simulink model "Lab4"  (R2022a)
settings: Solver=ode23t  StartTime=0.0  StopTime=3  MaxStep=1e-4  RelTol=1e-3
values from neighbouring files (symbols this model uses):
  f_1 = 50    [Lab4.m]
  J = 0.2    [Lab4.m]
  K2 = Lm/L2    (= 0.953488372093)    [Lab4.m]
  L_1 = L1*(1-K1*K2)    (= 0.0126279069767)    [Lab4.m]
  Llr = L2-Lm    (= 0.008)    [Lab4.m]
  Lls = L1-Lm    (= 0.005)    [Lab4.m]
  Pn = 5500    [Lab4.m]
  R1 = 1.32    [Lab4.m]
  R2 = 0.92    [Lab4.m]
  R_1 = (K2^2)*R2+R1    (= 2.15640886966)    [Lab4.m]
  T2 = L2/R2    (= 0.186956521739)    [Lab4.m]
  T_1 = L_1/R_1    (= 0.00585598916533)    [Lab4.m]
  Tn = Pn*z/((1-s_n)*2*pi*f_1)    (= 36.2840284769)    [Lab4.m]
  U_l = sqrt(3)*U_m    [Lab4.m]
  U_m = 220    [Lab4.m]
  w0 = 2*pi*f_1/z    (= 157.079632679)    [Lab4.m]
  z = 2    [Lab4.m]
libraries: mcbcontrolslib x4, spsControlledVoltageSourceLib x3, autolibim x2, spsAsynchronousMachineSIUnitsLib x1, spsGroundLib x1, spsThreePhaseVIMeasurementLib x1, simulink x1, spspowerguiLib x1
settings Model: Creator=hdu  LastModifiedBy=81502

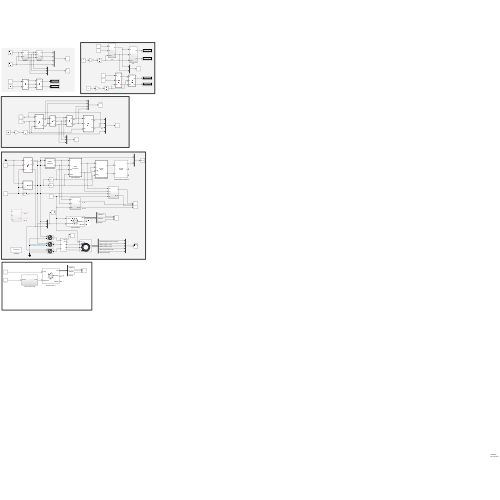
[thumbnail: Simulink's stored preview of the top-level diagram]
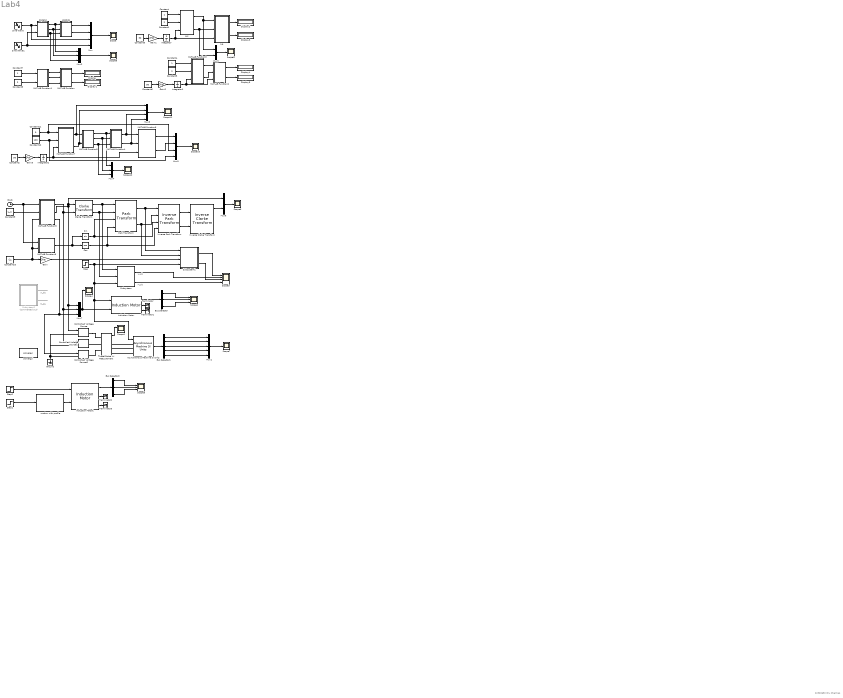
== system Lab4 ==
  note: 22320630
      | Zhu Chenhao
  note: w_ab
  note: M_ab
  note: w_dq
  note: M_dq
  Asynchronous Machine SI Units : spsAsynchronousMachineSIUnitsLib/Asynchronous Machine SI Units  RotorType=Squirrel-cage  PresetModel=No  MechanicalLoad=Torque Tm  ShowDetailedParameters=on  ReferenceFrame=Stationary  Units=SI  MeasurementBus=off  NominalParameters=[Pn U_l f_1]  VoltageRatio=1  Stator=[R1 Lls]  Rotor=[R2 Llr]  Cage1=[0.4155 0.002066]  Cage2=[0.4168 0.0003495]  Lm=Lm  Mechanical=[J 0.005752 z]  PolePairs=2  InitialConditions=[1 0 0 0 0 0 0 0]  SimulateSaturation=off  Saturation=[14.03593122, 27.81365428, 53.79336849, 72.68890987, 97.98006896, 148.6815601, 215.7428561, 302.9841135, 428.7778367 ; 230, 322, 414, 460, 506, 552, 598, 644, 690]  LoadFlowParameters=1492000  TsPowergui=0  TsBlock=-1  IterativeModel=Trapezoidal non iterative  IterativeDiscreteModel=Trapezoidal non iterative  Pmec=0
  Bus Selector : BusSelector  OutputSignals=IaStator,MtrSpd,MtrTrq
  Bus Selector1 : BusSelector  OutputSignals=Mechanical.Electromagnetic torque Te (N*m),Stator measurements.Stator current is_b (A),Stator measurements.Stator current is_a (A),Mechanical.Rotor angle thetam (rad),Mechanical.Rotor speed (wm)
  Bus Selector2 : BusSelector  OutputSignals=IaStator,MtrSpd,MtrTrq
  Clarke Transform : mcbcontrolslib/Clarke Transform  VariantControl=Variant2
  Clock : Clock
  Constant : Constant
  Constant1 : Constant  Value=2
  Constant10 : Constant  Value=f_1
  Constant11 : Constant  Value=0
  Constant12 : Constant  Value=100
  Constant2 : Constant  Value=50
  Constant3 : Constant  Value=50
  Constant4 : Constant
  Constant5 : Constant  Value=2
  Constant6 : Constant  Value=50
  Constant7 : Constant
  Constant8 : Constant  Value=2
  Constant9 : Constant  Value=U_m
  Controlled Voltage Source : spsControlledVoltageSourceLib/Controlled Voltage Source  Initialize=off  Source_Type=AC  Amplitude=0  Phase=0  Frequency=0  Measurements=None
  Controlled Voltage Source1 : spsControlledVoltageSourceLib/Controlled Voltage Source  Initialize=off  Source_Type=AC  Amplitude=0  Phase=0  Frequency=0  Measurements=None
  Controlled Voltage Source2 : spsControlledVoltageSourceLib/Controlled Voltage Source  Initialize=off  Source_Type=AC  Amplitude=0  Phase=0  Frequency=0  Measurements=None
  Cos : Trigonometry  Operator=cos
  Display{,1..5} (6 alike) : Display
  Gain{,1..3} (4 alike) : Gain  Gain=2*pi
  Ground : spsGroundLib/Ground  LConnTagsString=a
  Induction Motor : autolibim/Induction Motor  sim_type=Continuous  Ts=0.001  port_config=Torque  P=z  Zs=[R1 Lls]  Zr=[R2 Llr]  Lm=Lm  mechanical=[J 0 0]  theta_init=0  omega_init=0  RefBlkName='autolibim/Induction Motor'  aMode=1
      settings: SourceProductBaseCode=PW,DR,MT,VE
  Induction Motor1 : autolibim/Induction Motor  sim_type=Continuous  Ts=0.001  port_config=Torque  P=z  Zs=[R1 Lls]  Zr=[R2 Llr]  Lm=Lm  mechanical=[J 0 0]  theta_init=0  omega_init=0  RefBlkName='autolibim/Induction Motor'  aMode=1
      settings: SourceProductBaseCode=PW,DR,MT,VE
  Integrator : Integrator
  Integrator1 : Integrator
  Integrator2 : Integrator
  Inverse Clarke Transform : mcbcontrolslib/Inverse Clarke Transform
      settings: SourceProductBaseCode=MT
  Inverse Park Transform : mcbcontrolslib/Inverse Park Transform  AxisAlignment=D-axis
  MATLAB Function : MATLAB Function  TreatAsAtomicUnit=on
  MATLAB Function1 : MATLAB Function  TreatAsAtomicUnit=on
  MATLAB Function2 : MATLAB Function  TreatAsAtomicUnit=on
  MATLAB Function3 : MATLAB Function  TreatAsAtomicUnit=on
  MATLAB Function4 : MATLAB Function  TreatAsAtomicUnit=on
  MATLAB Function5 : MATLAB Function  TreatAsAtomicUnit=on
  MATLAB Function6 : MATLAB Function  TreatAsAtomicUnit=on
  MATLAB Function7 : MATLAB Function  TreatAsAtomicUnit=on
  MATLAB Function8 : MATLAB Function  TreatAsAtomicUnit=on
  MATLAB Function9 : MATLAB Function  TreatAsAtomicUnit=on
  Mux : Mux
  Mux1 : Mux  Inputs=5
  Mux2 : Mux  Inputs=3
  Mux3 : Mux  Inputs=2
  Mux4 : Mux  Inputs=3
  Mux5 : Mux
  Mux6 : Mux  Inputs=2
  Mux7 : Mux  Inputs=3
  Mux8 : Mux
  Park Transform : mcbcontrolslib/Park Transform  AxisAlignment=D-axis
      settings: SourceProductBaseCode=MT
  Scope{,4,6..12} (9 alike) : Scope
  Scope1 : Scope  NumInputPorts=2
  Scope2 : Scope  NumInputPorts=3
  Scope3 : Scope  NumInputPorts=4
  Scope5 : Scope  NumInputPorts=3
  Sin : Trigonometry
  Sine Wave : Sin  Amplitude=310  Frequency=2*pi*50  SampleTime=0
  Sine Wave1 : Sin  Amplitude=310  Frequency=2*pi*50  Phase=pi/2  SampleTime=0
  Step : Step  After=Tn  SampleTime=0
  Step1 : Step  Time=0.1  After=200  SampleTime=0
  Step2 : Step  Time=3  After=Tn  SampleTime=0
  Subsystem : Subsystem
  Subsystem1 : Subsystem
  Subsystem2 : Subsystem  Commented=on
  Terminator{,1..3} (4 alike) : Terminator
  Three-Phase V-I Measurement : spsThreePhaseVIMeasurementLib/Three-Phase V-I Measurement  VoltageMeasurement=phase-to-ground  SetLabelV=off  LabelV=Vabc  Vpu=off  VpuLL=off  CurrentMeasurement=yes  SetLabelI=off  LabelI=Iabc  Ipu=off  Pbase=100e6  Vbase=500e3  OutputType=Complex  PhasorSimulation=off  PSBequivalent=0
  abc2dp : Subsystem
  dq2abc : Subsystem
  e-s : Subsystem
  motion with profile : Subsystem
  powergui : spspowerguiLib/powergui  Priority=1  SimulationMode=Continuous  SampleTime=50e-6  frequency=60  Iterations=50  frequencyindice=50  Pbase=100e6  ErrMax=1e-4  UnitsV=kV  UnitsW=MW  buscounter=0  FunctionMessages=off  echomessages=off  EnableUseOfTLC=off  CurrentSourceSwitches=off  DisableSnubberDevices=off  DisableRonSwitches=off  DisableVfSwitches=off  DisplayEquations=off  AutomaticDiscreteSolvers=off  SolverType=Tustin/Backward Euler (TBE)  Interpol=off  ExternalGateDelay=off  methode=off  Ts=100  x0status=blocks  SPID=on  SwTol=0  HookPort=off  NonlinearTolerance=1e-4  nMaxIteration=100  ContinueOnMaxIteration=off  RestoreLinks=warning  ResistiveCurrentMeasurement=off  Frange=[0:2:500]  Ylog=off  Xlog=on  ShowGrid=off  save=off  variable=ZData  structure=0  ZoomFFT=off  StartTime=0.0  cycles=1  DisplayStyle=1  fundamental=60  FreqAxis=off  MaxFrequency=1000  frequencyindicesteady=1  RmsSteady=1  display=off
  s-e : Subsystem
  wires:
  Constant10/1 -> MATLAB Function9/3(f_1), MATLAB Function8/2(f_1), Gain/1
  Clock/1 -> MATLAB Function8/1(t), MATLAB Function9/1(t)
  MATLAB Function8/1(theta) -> Sin/1, Cos/1
  Constant9/1 -> MATLAB Function9/2(A)
  MATLAB Function9/2(ub) -> Mux6/1, Clarke Transform/1, Controlled Voltage Source/1, Mux7/1
  MATLAB Function9/1(ua) -> Clarke Transform/2, Mux7/2, Controlled Voltage Source1/1
  Clarke Transform/1 -> Park Transform/1, Subsystem/1(Ua)
  Clarke Transform/2 -> Subsystem/2(Ub), Park Transform/2
  Sin/1 -> Park Transform/3, Inverse Park Transform/3
  Cos/1 -> Park Transform/4, Inverse Park Transform/4
  Park Transform/2 -> Inverse Park Transform/2, Subsystem1/2(Uq)
  Park Transform/1 -> Inverse Park Transform/1, Subsystem1/1(Ud)
  Step/1 -> Asynchronous Machine SI Units/1, Induction Motor/1, Subsystem/3(Mc), Subsystem1/4(Mc)
  Inverse Park Transform/2 -> Inverse Clarke Transform/2
  Inverse Park Transform/1 -> Inverse Clarke Transform/1
  Inverse Clarke Transform/1 -> Mux6/2
  MATLAB Function9/3(uc) -> Controlled Voltage Source2/1, Mux7/3
  Mux7/1 -> Scope4/1, Induction Motor/2
  Mux6/1 -> Scope6/1
  Induction Motor/2 -> Terminator/1
  Induction Motor/1 -> Bus Selector/1
  Bus Selector/1 -> Scope2/1  "<IaStator>"
  Bus Selector/2 -> Scope2/2  "<MtrSpd>"
  Bus Selector/3 -> Scope2/3  "<MtrTrq>"
  Subsystem/1(w) -> Scope3/2
  Subsystem/2(M din) -> Scope3/4
  Asynchronous Machine SI Units/1 -> Bus Selector1/1
  Bus Selector1/1 -> Mux1/1  "<Electromagnetic torque Te (N*m)>"
  Bus Selector1/3 -> Mux1/3  "<Stator current is_a (A)>"
  Bus Selector1/4 -> Mux1/4  "<Rotor angle thetam (rad)>"
  Bus Selector1/5 -> Mux1/5  "<Rotor speed (wm)>"
  Bus Selector1/2 -> Mux1/2  "<Stator current is_b (A)>"
  Mux1/1 -> Scope7/1
  Gain/1 -> Subsystem1/3(w1)
  Subsystem1/1(w) -> Scope3/1
  Subsystem1/2(M din) -> Scope3/3
  Three-Phase V-I Measurement/1 -> Scope1/1
  Subsystem2/2(M din) -> ?
  Subsystem2/1(w) -> ?
  Induction Motor/3 -> Terminator1/1
  Induction Motor1/3 -> Terminator3/1
  Bus Selector2/3 -> Scope5/3  "<MtrTrq>"
  Induction Motor1/2 -> Terminator2/1
  Induction Motor1/1 -> Bus Selector2/1
  Bus Selector2/1 -> Scope5/1  "<IaStator>"
  Bus Selector2/2 -> Scope5/2  "<MtrSpd>"
  Step2/1 -> Induction Motor1/1
  Mux5/1 -> Scope10/1
  Constant6/1 -> Gain2/1
  Constant2/1 -> Gain3/1
  e-s/2(qs) -> Mux3/2, s-e/2(qs)
  Mux2/1 -> Scope8/1
  Mux8/1 -> Scope11/1
  Constant4/1 -> MATLAB Function3/1(de)
  Gain3/1 -> Integrator2/1
  MATLAB Function6/1(de) -> Mux5/1  "de"
  MATLAB Function7/2(qs) -> Mux8/2, MATLAB Function5/2(qs)  "qs"
  MATLAB Function1/1(a) -> MATLAB Function/1(a)
  e-s/1(ds) -> Mux3/1, s-e/1(ds)
  Constant3/1 -> Gain1/1
  MATLAB Function4/2(qs) -> Mux8/4, MATLAB Function6/2(qs)  "qs1"
  Mux3/1 -> Scope9/1
  MATLAB Function7/1(ds) -> Mux8/1, MATLAB Function5/1(ds)  "ds"
  MATLAB Function4/1(ds) -> Mux8/3, MATLAB Function6/1(ds)  "ds1"
  Integrator/1 -> s-e/3(theta), e-s/3(theta)
  Constant11/1 -> Mux5/3, MATLAB Function7/1(de)  "de"
  MATLAB Function3/1(ds) -> MATLAB Function2/1(ds)
  dq2abc/3(c) -> abc2dp/3(c), Mux2/3
  Mux4/1 -> Scope12/1
  abc2dp/2(qs) -> Mux/2
  MATLAB Function/2(qs) -> Display1/1
  Constant7/1 -> MATLAB Function1/1(ds)
  MATLAB Function1/3(c) -> MATLAB Function/3(c)
  Constant8/1 -> MATLAB Function1/2(qs)
  Sine Wave1/1 -> dq2abc/2(qs), Mux/4
  Integrator1/1 -> MATLAB Function2/3(teta), MATLAB Function3/3(teta)
  MATLAB Function2/2(qe) -> Display5/1
  MATLAB Function3/2(qs) -> MATLAB Function2/2(qs)
  Constant12/1 -> Mux5/4, MATLAB Function7/2(qe)  "qe"
  MATLAB Function1/2(b) -> MATLAB Function/2(b)
  Gain2/1 -> Integrator1/1
  MATLAB Function6/2(qe) -> Mux5/2  "dq"
  Gain1/1 -> Integrator/1
  MATLAB Function5/2(b) -> Mux4/2, MATLAB Function4/2(b)  "b"
  Mux/1 -> Scope/1
  s-e/2(qe) -> Display3/1
  MATLAB Function5/1(a) -> Mux4/1, MATLAB Function4/1(a)  "a"
  Integrator2/1 -> MATLAB Function6/3(teta), MATLAB Function7/3(teta)
  s-e/1(de) -> Display2/1
  Constant1/1 -> e-s/2(qe)
  Sine Wave/1 -> Mux/3, dq2abc/1(ds)
  MATLAB Function/1(ds) -> Display/1
  Constant/1 -> e-s/1(de)
  MATLAB Function2/1(de) -> Display4/1
  abc2dp/1(ds) -> Mux/1
  Constant5/1 -> MATLAB Function3/2(qe)
  dq2abc/1(a) -> Mux2/1, abc2dp/1(a)
  MATLAB Function5/3(c) -> Mux4/3, MATLAB Function4/3(c)  "c"
  dq2abc/2(b) -> Mux2/2, abc2dp/2(b)
  Step1/1 -> motion with profile/1(Speed)
  motion with profile/1(Vabc) -> Induction Motor1/2
  connections:
  Ground/LConn1 -- Controlled Voltage Source/LConn1 -- Controlled Voltage Source1/LConn1 -- Controlled Voltage Source2/LConn1
  Three-Phase V-I Measurement/LConn2 -- Controlled Voltage Source1/RConn1
  Controlled Voltage Source/RConn1 -- Three-Phase V-I Measurement/LConn1
  Three-Phase V-I Measurement/LConn3 -- Controlled Voltage Source2/RConn1
  Asynchronous Machine SI Units/LConn1 -- Three-Phase V-I Measurement/RConn1
  Asynchronous Machine SI Units/LConn2 -- Three-Phase V-I Measurement/RConn2
  Asynchronous Machine SI Units/LConn3 -- Three-Phase V-I Measurement/RConn3

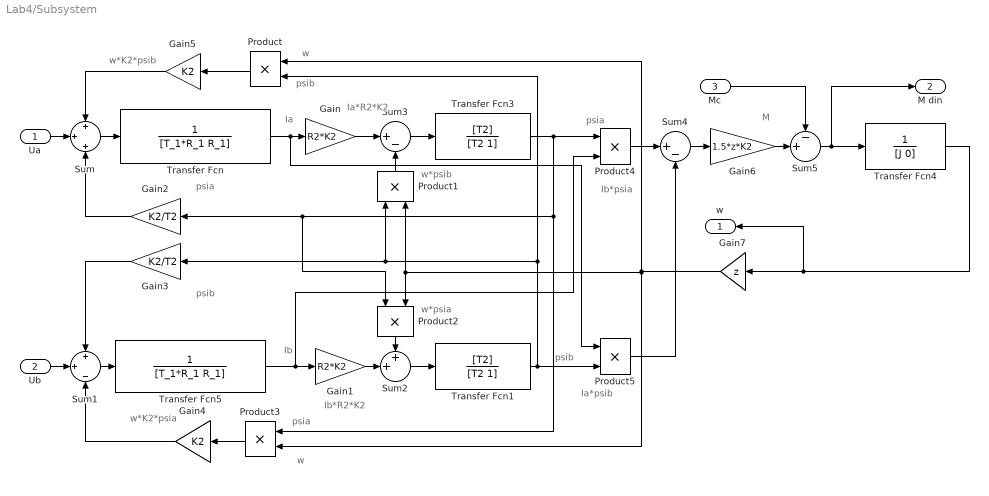
== system Lab4/Subsystem ==
  note: Ia*psib
  note: psib
  note: w
  note: psia
  note: w
  note: psib
  note: w*psia
  note: M
  note: Ib*psia
  note: psia
  note: w*psib
  note: Ib
  note: psib
  note: psia
  note: Ia
  note: w*K2*psib
  note: w*K2*psia
  note: Ia*R2*K2
  note: Ib*R2*K2
  Ua : Inport
  Ub : Inport  Port=2
  Mc : Inport  Port=3
  Gain : Gain  Gain=R2*K2
  Gain1 : Gain  Gain=R2*K2
  Gain2 : Gain  Gain=K2/T2
  Gain3 : Gain  Gain=K2/T2
  Gain4 : Gain  Gain=K2
  Gain5 : Gain  Gain=K2
  Gain6 : Gain  Gain=1.5*z*K2
  Gain7 : Gain  Gain=z
  Product{,1..5} (6 alike) : Product
  Sum : Sum  Inputs=+|+|+
  Sum1 : Sum  Inputs=+|+|-
  Sum2 : Sum  Inputs=++|
  Sum3 : Sum  Inputs=|+-
  Sum4 : Sum  Inputs=|+-
  Sum5 : Sum  Inputs=-+|
  Transfer Fcn : TransferFcn  Denominator=[T_1*R_1 R_1]
  Transfer Fcn1 : TransferFcn  Numerator=[T2]  Denominator=[T2 1]
  Transfer Fcn3 : TransferFcn  Numerator=[T2]  Denominator=[T2 1]
  Transfer Fcn4 : TransferFcn  Denominator=[J 0]
  Transfer Fcn5 : TransferFcn  Denominator=[T_1*R_1 R_1]
  w : Outport  VectorParamsAs1DForOutWhenUnconnected=off
  M din : Outport  Port=2  VectorParamsAs1DForOutWhenUnconnected=off
  wires:
  Transfer Fcn5/1 -> Gain1/1, Product4/2
  Product4/1 -> Sum4/1
  Product2/1 -> Sum2/1
  Sum3/1 -> Transfer Fcn3/1
  Gain5/1 -> Sum/1
  Sum/1 -> Transfer Fcn/1
  Sum5/1 -> M din/1, Transfer Fcn4/1
  Gain6/1 -> Sum5/2
  Gain2/1 -> Sum/3
  Product5/1 -> Sum4/2
  Gain7/1 -> Product3/2, Product1/2, Product2/2, Product/1
  Product1/1 -> Sum3/2
  Transfer Fcn/1 -> Product5/1, Gain/1
  Transfer Fcn1/1 -> Product5/2, Product/2, Product1/1, Gain3/1
  Gain3/1 -> Sum1/1
  Gain/1 -> Sum3/1
  Transfer Fcn4/1 -> w/1, Gain7/1
  Mc/1 -> Sum5/1
  Sum4/1 -> Gain6/1
  Gain1/1 -> Sum2/2
  Gain4/1 -> Sum1/3
  Sum1/1 -> Transfer Fcn5/1
  Product/1 -> Gain5/1
  Sum2/1 -> Transfer Fcn1/1
  Product3/1 -> Gain4/1
  Ua/1 -> Sum/2
  Transfer Fcn3/1 -> Product4/1, Product3/1, Product2/1, Gain2/1
  Ub/1 -> Sum1/2

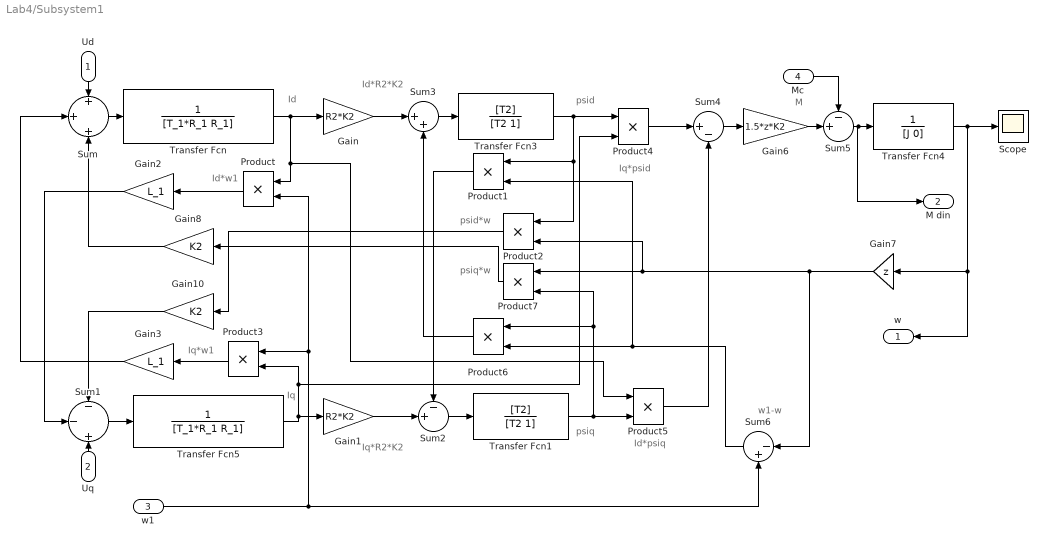
== system Lab4/Subsystem1 ==
  note: w1-w
  note: psiq*w
  note: Iq*w1
  note: Id*psiq
  note: psiq
  note: M
  note: Iq*psid
  note: psid
  note: Iq
  note: Id
  note: Id*R2*K2
  note: Iq*R2*K2
  note: Id*w1
  note: psid*w
  Ud : Inport
  Uq : Inport  Port=2
  w1 : Inport  Port=3
  Mc : Inport  Port=4
  Gain : Gain  Gain=R2*K2
  Gain1 : Gain  Gain=R2*K2
  Gain10 : Gain  Gain=K2
  Gain2 : Gain  Gain=L_1
  Gain3 : Gain  Gain=L_1
  Gain6 : Gain  Gain=1.5*z*K2
  Gain7 : Gain  Gain=z
  Gain8 : Gain  Gain=K2
  Product{,1..7} (8 alike) : Product
  Scope : Scope
  Sum : Sum  Inputs=+|+|+
  Sum1 : Sum  Inputs=-|-|+
  Sum2 : Sum  Inputs=-+|
  Sum3 : Sum  Inputs=|++
  Sum4 : Sum  Inputs=|+-
  Sum5 : Sum  Inputs=-+|
  Sum6 : Sum  Inputs=|-+
  Transfer Fcn : TransferFcn  Denominator=[T_1*R_1 R_1]
  Transfer Fcn1 : TransferFcn  Numerator=[T2]  Denominator=[T2 1]
  Transfer Fcn3 : TransferFcn  Numerator=[T2]  Denominator=[T2 1]
  Transfer Fcn4 : TransferFcn  Denominator=[J 0]
  Transfer Fcn5 : TransferFcn  Denominator=[T_1*R_1 R_1]
  w : Outport  VectorParamsAs1DForOutWhenUnconnected=off
  M din : Outport  Port=2  VectorParamsAs1DForOutWhenUnconnected=off
  wires:
  Sum/1 -> Transfer Fcn/1
  Sum5/1 -> M din/1, Transfer Fcn4/1
  Gain6/1 -> Sum5/2
  Mc/1 -> Sum5/1
  Gain1/1 -> Sum2/2
  Sum1/1 -> Transfer Fcn5/1
  Transfer Fcn1/1 -> Product7/2, Product6/1, Product5/2
  Transfer Fcn/1 -> Product5/1, Product/1, Gain/1
  Gain/1 -> Sum3/1
  Sum3/1 -> Transfer Fcn3/1
  Product4/1 -> Sum4/1
  Sum4/1 -> Gain6/1
  Product/1 -> Gain2/1
  Uq/1 -> Sum1/3
  Gain2/1 -> Sum1/2
  Transfer Fcn3/1 -> Product4/1, Product2/1, Product1/1
  Product6/1 -> Sum3/2
  Product1/1 -> Sum2/1
  Product7/1 -> Gain8/1
  Product2/1 -> Gain10/1
  Gain8/1 -> Sum/3
  Gain10/1 -> Sum1/1
  Transfer Fcn5/1 -> Product4/2, Product3/2, Gain1/1
  Sum2/1 -> Transfer Fcn1/1
  Product5/1 -> Sum4/2
  Product3/1 -> Gain3/1
  Transfer Fcn4/1 -> Scope/1, w/1, Gain7/1
  Gain7/1 -> Product7/1, Product2/2, Sum6/1
  Sum6/1 -> Product1/2, Product6/2
  w1/1 -> Product3/1, Product/2, Sum6/2
  Ud/1 -> Sum/1
  Gain3/1 -> Sum/2

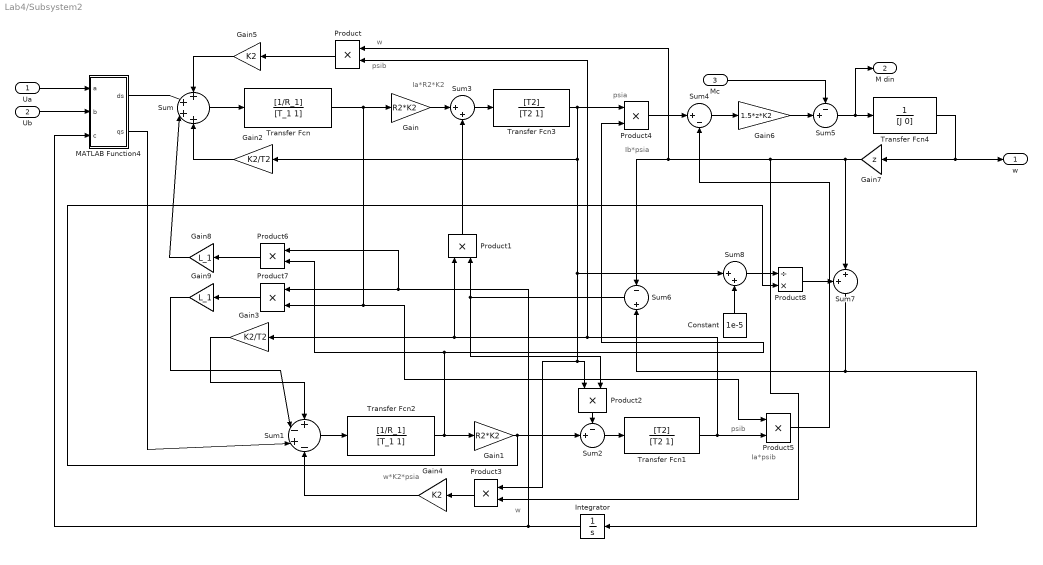
== system Lab4/Subsystem2 ==
  note: Ia*psib
  note: psib
  note: w
  note: w
  note: psib
  note: Ib*psia
  note: psia
  note: w*K2*psia
  note: Ia*R2*K2
  Ua : Inport
  Ub : Inport  Port=2
  Mc : Inport  Port=3
  Constant : Constant  Value=1e-5
  Gain : Gain  Gain=R2*K2
  Gain1 : Gain  Gain=R2*K2
  Gain2 : Gain  Gain=K2/T2
  Gain3 : Gain  Gain=K2/T2
  Gain4 : Gain  Gain=K2
  Gain5 : Gain  Gain=K2
  Gain6 : Gain  Gain=1.5*z*K2
  Gain7 : Gain  Gain=z
  Gain8 : Gain  Gain=L_1
  Gain9 : Gain  Gain=L_1
  Integrator : Integrator
  MATLAB Function4 : MATLAB Function  TreatAsAtomicUnit=on
  Product{,1..7} (8 alike) : Product
  Product8 : Product  Inputs=/*
  Sum : Sum  Inputs=+|+|+|+
  Sum1 : Sum  Inputs=+|-|+|-
  Sum2 : Sum  Inputs=-+|
  Sum3 : Sum  Inputs=|++
  Sum4 : Sum  Inputs=|+-
  Sum5 : Sum  Inputs=-+|
  Sum6 : Sum  Inputs=-+
  Sum7 : Sum  Inputs=++|
  Sum8 : Sum  Inputs=|++
  Transfer Fcn : TransferFcn  Numerator=[1/R_1]  Denominator=[T_1 1]
  Transfer Fcn1 : TransferFcn  Numerator=[T2]  Denominator=[T2 1]
  Transfer Fcn2 : TransferFcn  Numerator=[1/R_1]  Denominator=[T_1 1]
  Transfer Fcn3 : TransferFcn  Numerator=[T2]  Denominator=[T2 1]
  Transfer Fcn4 : TransferFcn  Denominator=[J 0]
  w : Outport  VectorParamsAs1DForOutWhenUnconnected=off
  M din : Outport  Port=2  VectorParamsAs1DForOutWhenUnconnected=off
  wires:
  Sum1/1 -> Transfer Fcn2/1
  Product4/1 -> Sum4/1
  Product2/1 -> Sum2/1
  Sum3/1 -> Transfer Fcn3/1
  Gain5/1 -> Sum/1
  Sum/1 -> Transfer Fcn/1
  Sum5/1 -> M din/1, Transfer Fcn4/1
  Gain6/1 -> Sum5/2
  Gain2/1 -> Sum/4
  Product5/1 -> Sum4/2
  Gain7/1 -> Sum6/1, Product/1, Product3/2, Sum7/2
  Product1/1 -> Sum3/2
  Transfer Fcn/1 -> Gain/1, Product5/1, Product7/2
  Transfer Fcn1/1 -> Product5/2, Gain3/1, Product1/1, Product/2
  Gain3/1 -> Sum1/1
  Gain/1 -> Sum3/1
  Transfer Fcn4/1 -> Gain7/1, w/1
  Mc/1 -> Sum5/1
  Sum4/1 -> Gain6/1
  Gain1/1 -> Sum2/2, Product8/2
  Gain4/1 -> Sum1/4
  Product/1 -> Gain5/1
  Sum2/1 -> Transfer Fcn1/1
  Product3/1 -> Gain4/1
  Transfer Fcn3/1 -> Gain2/1, Product3/1, Product2/1, Sum8/1, Product4/1
  Product6/1 -> Gain8/1
  Product7/1 -> Gain9/1
  Ua/1 -> MATLAB Function4/1(a)
  Ub/1 -> MATLAB Function4/2(b)
  MATLAB Function4/1(ds) -> Sum/2
  Gain8/1 -> Sum/3
  Transfer Fcn2/1 -> Gain1/1, Product6/2, Product4/2
  Sum6/1 -> Product1/2, Product2/2
  Product8/1 -> Sum7/1
  Sum8/1 -> Product8/1
  Constant/1 -> Sum8/2
  Integrator/1 -> Product6/1, Product7/1, MATLAB Function4/3(c)
  Sum7/1 -> Sum6/2, Integrator/1
  Gain9/1 -> Sum1/2
  MATLAB Function4/2(qs) -> Sum1/3

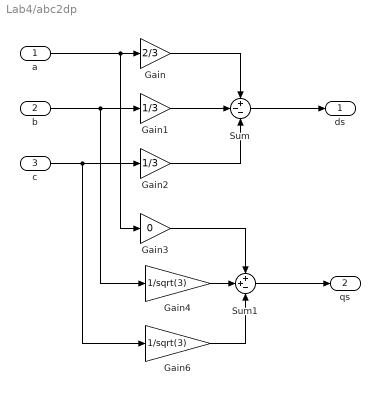
== system Lab4/abc2dp ==
  a : Inport
  b : Inport  Port=2
  c : Inport  Port=3
  Gain : Gain  Gain=2/3
  Gain1 : Gain  Gain=1/3
  Gain2 : Gain  Gain=1/3
  Gain3 : Gain  Gain=0
  Gain4 : Gain  Gain=1/sqrt(3)
  Gain6 : Gain  Gain=1/sqrt(3)
  Sum : Sum  Inputs=+--
  Sum1 : Sum  Inputs=++-
  ds : Outport
  qs : Outport  Port=2
  wires:
  b/1 -> Gain4/1, Gain1/1
  a/1 -> Gain3/1, Gain/1
  c/1 -> Gain6/1, Gain2/1
  Gain4/1 -> Sum1/2
  Gain3/1 -> Sum1/1
  Gain1/1 -> Sum/2
  Gain/1 -> Sum/1
  Sum1/1 -> qs/1
  Gain6/1 -> Sum1/3
  Sum/1 -> ds/1
  Gain2/1 -> Sum/3

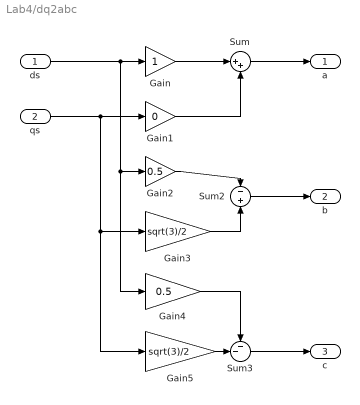
== system Lab4/dq2abc ==
  ds : Inport
  qs : Inport  Port=2
  Gain : Gain
  Gain1 : Gain  Gain=0
  Gain2 : Gain  Gain=0.5
  Gain3 : Gain  Gain=sqrt(3)/2
  Gain4 : Gain  Gain=0.5
  Gain5 : Gain  Gain=sqrt(3)/2
  Sum : Sum  Inputs=|++
  Sum2 : Sum  Inputs=-+
  Sum3 : Sum  Inputs=--|
  a : Outport
  b : Outport  Port=2
  c : Outport  Port=3
  wires:
  ds/1 -> Gain4/1, Gain2/1, Gain/1
  qs/1 -> Gain3/1, Gain5/1, Gain1/1
  Gain1/1 -> Sum/2
  Gain/1 -> Sum/1
  Sum/1 -> a/1
  Gain5/1 -> Sum3/2
  Gain4/1 -> Sum3/1
  Gain3/1 -> Sum2/2
  Gain2/1 -> Sum2/1
  Sum2/1 -> b/1
  Sum3/1 -> c/1

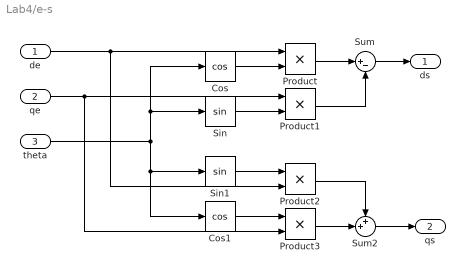
== system Lab4/e-s ==
  de : Inport
  qe : Inport  Port=2
  theta : Inport  Port=3
  Cos : Trigonometry  Operator=cos
  Cos1 : Trigonometry  Operator=cos
  Product{,1..3} (4 alike) : Product
  Sin : Trigonometry
  Sin1 : Trigonometry
  Sum : Sum  Inputs=|+-
  Sum2 : Sum  Inputs=++|
  ds : Outport
  qs : Outport  Port=2
  wires:
  de/1 -> Product/1, Product2/2
  qe/1 -> Product3/2, Product1/1
  Sum/1 -> ds/1
  Sum2/1 -> qs/1
  Cos/1 -> Product/2
  Sin/1 -> Product1/2
  Sin1/1 -> Product2/1
  Cos1/1 -> Product3/1
  theta/1 -> Cos/1, Sin/1, Cos1/1, Sin1/1
  Product/1 -> Sum/1
  Product3/1 -> Sum2/2
  Product2/1 -> Sum2/1
  Product1/1 -> Sum/2

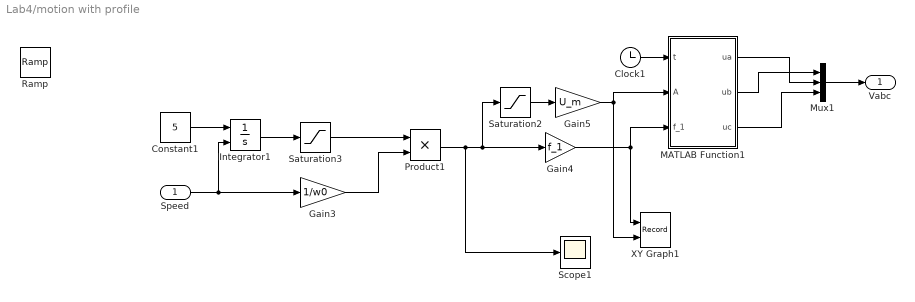
== system Lab4/motion with profile ==
  Speed : Inport
  Clock1 : Clock
  Constant1 : Constant  Value=5
  Gain3 : Gain  Gain=1/w0
  Gain4 : Gain  Gain=f_1
  Gain5 : Gain  Gain=U_m
  Integrator1 : Integrator  ExternalReset=rising
  MATLAB Function1 : MATLAB Function  TreatAsAtomicUnit=on
  Mux1 : Mux  Inputs=3
  Product1 : Product
  Ramp : simulink/Sources/Ramp  slope=1  start=0  InitialOutput=0
  Saturation2 : Saturate  UpperLimit=1  LowerLimit=0.1
  Saturation3 : Saturate  UpperLimit=1  LowerLimit=0
  Scope1 : Scope
  XY Graph1 : Record  FileSettingsInternal="{\"entries\":[{\"content\":{\"excelSettings\":{\"content\":{},\"type\":\"Streamout.ExcelSettings\"}},\"type\":\"Streamout.FileSettingStorage\",\"uuid\":\"99df4d59-c83d-4dc5-a817-25199a01b009\"}],\"packageUris\":[\"http://schema.mathworks.com/mf0/streamout_blocks/R2020a\"],\"version\":\"1.0\"}"  Layout=[1 1]  SignalsInternal="{\"entries\":[{\"content\":{\"signals\":[{\"content\":{\"blockPath\":[\"Lab4_end/motion with profile/XY Graph1\"],\"channel\":[],\"dimensions\":[1],\"domain\":\"Lab4_end/motion with profile/XY Graph1\",\"lineColor\":\"#a2142f\",\"plots\":[1],\"port\":1,\"sid\":[\"\"],\"signalID\":822,\"signalName\":\"Gain4\"},\"type\":\"RecordBlkView.Signal\",\"uuid\":\"4c821ef0-3557-4c55-9368-60d8e7b24f6e\"},{\"content\":{\"blockPath\":[\"Lab4_end/motion with profile/XY Graph1\"],\"channel\":[],\"dimensions\":[1],\"domain\":\"Lab4_end/motion with profile/XY Graph1\",\"lineColor\":\"#139fff\",\"plots\":[1],\"port\":2,\"sid\":[\"\"],\"signalID\":826,\"signalName\":\"Gain5\"},\"type\":\"RecordBlkView.Signal\",\"uuid\":\"d8a737b0-6d68-461f-91d3-654044413d69\"}]},\"type\":\"RecordBlkView.InputSignals\",\"uuid\":\"a021e36a-3f52-44ee-b583-821890dc44ac\"}],\"packageUris\":[\"http://schema.mathworks.com/mf0/streamout_blocks/R2020a\"],\"version\":\"1.0\"}"  VisualizationBindings="{\"xyplotplugin\":{\"info\":[{\"series\":[{\"bindingParametersList\":[{\"parameter\":\"X-Axis\",\"signalID\":822,\"signalName\":\"Gain4\"},{\"parameter\":\"Y-Axis\",\"signalID\":826,\"signalName\":\"Gain5\"}],\"seriesID\":62947}],\"subplotID\":1}]}}"  CompatibilityTag=XY  st=-1
  Vabc : Outport
  wires:
  Constant1/1 -> Integrator1/1
  Saturation3/1 -> Product1/1
  Integrator1/1 -> Saturation3/1
  Speed/1 -> Integrator1/2, Gain3/1
  MATLAB Function1/1(ua) -> Mux1/2
  Gain4/1 -> MATLAB Function1/3(f_1), XY Graph1/1
  Gain3/1 -> Product1/2
  Gain5/1 -> MATLAB Function1/2(A), XY Graph1/2
  Saturation2/1 -> Gain5/1
  MATLAB Function1/3(uc) -> Mux1/3
  Clock1/1 -> MATLAB Function1/1(t)
  Mux1/1 -> Vabc/1
  MATLAB Function1/2(ub) -> Mux1/1
  Product1/1 -> Scope1/1, Gain4/1, Saturation2/1

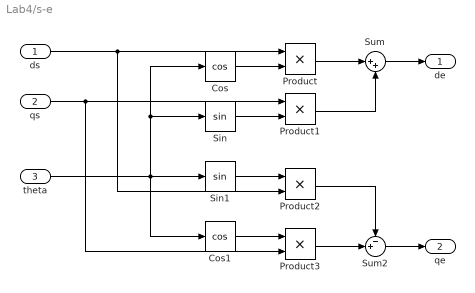
== system Lab4/s-e ==
  ds : Inport
  qs : Inport  Port=2
  theta : Inport  Port=3
  Cos : Trigonometry  Operator=cos
  Cos1 : Trigonometry  Operator=cos
  Product{,1..3} (4 alike) : Product
  Sin : Trigonometry
  Sin1 : Trigonometry
  Sum : Sum  Inputs=|++
  Sum2 : Sum  Inputs=-+|
  de : Outport
  qe : Outport  Port=2
  wires:
  ds/1 -> Product2/2, Product/1
  qs/1 -> Product3/2, Product1/1
  Sum/1 -> de/1
  Sum2/1 -> qe/1
  Cos/1 -> Product/2
  Sin/1 -> Product1/2
  Sin1/1 -> Product2/1
  Cos1/1 -> Product3/1
  theta/1 -> Cos/1, Sin/1, Cos1/1, Sin1/1
  Product/1 -> Sum/1
  Product3/1 -> Sum2/2
  Product2/1 -> Sum2/1
  Product1/1 -> Sum/2

== matlab function Lab4/MATLAB Function6 ==
  data: ds input; de output; qs input; teta input; qe output
function [de, qe] = fcn(ds, qs, teta)
    de = ds*cos(teta) + qs*sin(teta);
    qe = - ds*sin(teta) + qs*cos(teta);

== matlab function Lab4/MATLAB Function ==
  data: a input; ds output; b input; c input; qs output
function [ds,qs] = fcn(a,b,c)
    ds = (a*2/3) - (b/3) - (c/3);
    qs = (b/(sqrt(3))) - (c/(sqrt(3)));
    [ds; qs];

== matlab function Lab4/MATLAB Function7 ==
  data: de input; ds output; qe input; teta input; qs output
function [ds, qs] = fcn(de, qe, teta)
    ds = de*cos(teta) - qe*sin(teta);
    qs = de*sin(teta) + qe*cos(teta);

== matlab function Lab4/motion with profile/MATLAB Function1 ==
  data: t input; ua output; A input; f_1 input; ub output; uc output
function [ua, ub, uc] = fcn(t, A, f_1)
    ua = A*sin(2*pi*f_1*t);
    ub = A*sin(2*pi*f_1*t + 2/3*pi);
    uc = A*sin(2*pi*f_1*t - 2/3*pi);

== matlab function Lab4/MATLAB Function1 ==
  data: ds input; a output; qs input; b output; c output
function [a,b,c] = fcn(ds,qs)
    a = ds;
    b = -0.5*ds + qs*sqrt(3)/2;
    c = -0.5*ds - qs*sqrt(3)/2;
    [a,b,c];

== matlab function Lab4/MATLAB Function2 ==
  data: ds input; de output; qs input; teta input; qe output
function [de, qe] = fcn(ds, qs, teta)
    de = ds*cos(teta) + qs*sin(teta);
    qe = - ds*sin(teta) + qs*cos(teta);
    [de; qe];

== matlab function Lab4/Subsystem2/MATLAB Function4 ==
  data: a input; ds output; b input; c input; qs output
function [ds,qs] = fcn(a,b,c)
    ds = (a*2/3) - (b/3) - (c/3);
    qs = (b/(sqrt(3))) - (c/(sqrt(3)));

== matlab function Lab4/MATLAB Function3 ==
  data: de input; ds output; qe input; teta input; qs output
function [ds, qs] = fcn(de, qe, teta)
    ds = de*cos(teta) - qe*sin(teta);
    qs = de*sin(teta) + qe*cos(teta);
    [ds; qs];

== matlab function Lab4/MATLAB Function4 ==
  data: a input; ds output; b input; c input; qs output
function [ds,qs] = fcn(a,b,c)
    ds = (a*2/3) - (b/3) - (c/3);
    qs = (b/(sqrt(3))) - (c/(sqrt(3)));

== matlab function Lab4/MATLAB Function5 ==
  data: ds input; a output; qs input; b output; c output
function [a,b,c] = fcn(ds,qs)
    a = ds;
    b = -0.5*ds + qs*sqrt(3)/2;
    c = -0.5*ds - qs*sqrt(3)/2;

== matlab function Lab4/MATLAB Function8 ==
  data: t input; theta output; f_1 input
function theta  = fcn(t,f_1)
    theta = 2*t*pi*f_1;

== matlab function Lab4/MATLAB Function9 ==
  data: t input; ua output; A input; f_1 input; ub output; uc output
function [ua, ub, uc] = fcn(t, A, f_1)
    ua = A*sin(2*pi*f_1*t);
    ub = A*sin(2*pi*f_1*t + 2/3*pi);
    uc = A*sin(2*pi*f_1*t - 2/3*pi);
